simulink model "Monod_Controller"  (R2020b)
settings: Solver=FixedStepAuto  StartTime=0.0  StopTime=constants.tend  FixedStep=constants.dt  RelTol=1e-3
undefined symbols (not defined in the file or in its folder): constants
libraries: pid_lib x2
settings Model: Creator=newpo  LastModifiedBy=newpo
settings DataIOCC: ReturnWorkspaceOutputs=off

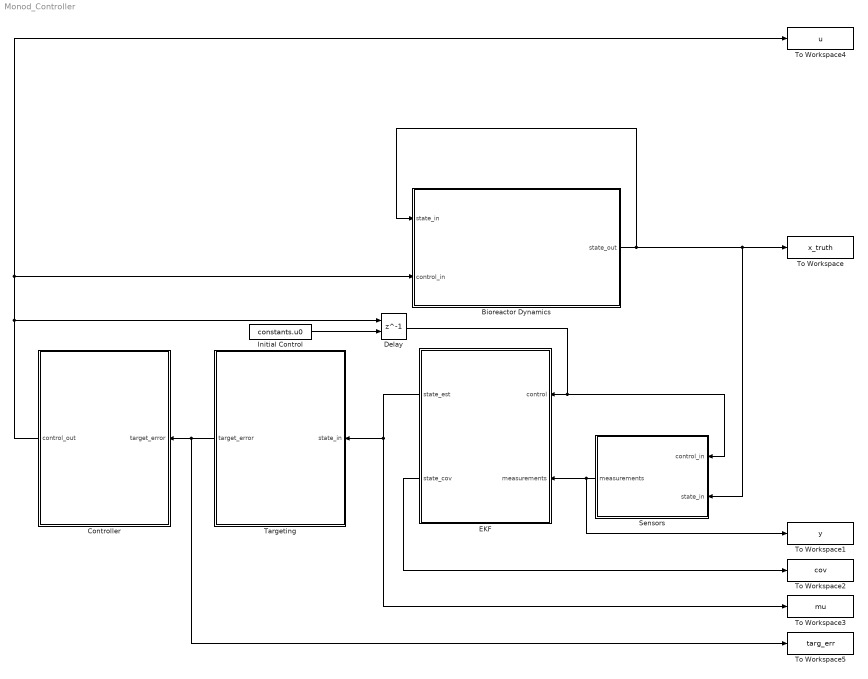
== system Monod_Controller ==
  Bioreactor Dynamics : Subsystem
  Controller : Subsystem
  Delay : Delay  DelayLength=1  InitialConditionSource=Input port  InitialCondition=[constants.w;0;0;constants.Fg]
      settings: InputPortMap=u0,p4
  EKF : Subsystem
  Initial Control : Constant  Value=constants.u0
  Sensors : Subsystem
  Targeting : Subsystem
  To Workspace : ToWorkspace  VariableName=x_truth  SampleTime=-1
  To Workspace1 : ToWorkspace  VariableName=y  SampleTime=-1
  To Workspace2 : ToWorkspace  VariableName=cov  SampleTime=-1
  To Workspace3 : ToWorkspace  VariableName=mu  SampleTime=-1
  To Workspace4 : ToWorkspace  VariableName=u  SampleTime=-1
  To Workspace5 : ToWorkspace  VariableName=targ_err  SampleTime=-1
  wires:
  Bioreactor Dynamics/1(state_out) -> Sensors/2(state_in), To Workspace/1, Bioreactor Dynamics/1(state_in)
  Sensors/1(measurements) -> To Workspace1/1, EKF/2(measurements)
  EKF/1(state_est) -> To Workspace3/1, Targeting/1(state_in)
  Controller/1(control_out) -> To Workspace4/1, Bioreactor Dynamics/2(control_in), Delay/1
  Targeting/1(target_error) -> To Workspace5/1, Controller/1(target_error)
  EKF/2(state_cov) -> To Workspace2/1
  Delay/1 -> Sensors/1(control_in), EKF/1(control)
  Initial Control/1 -> Delay/2

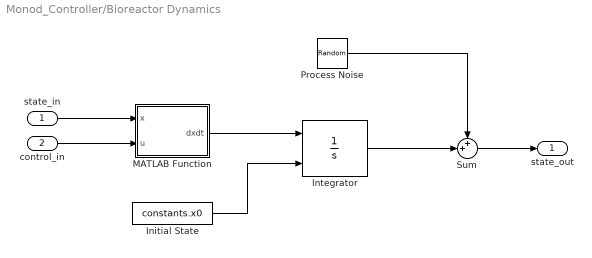
== system Monod_Controller/Bioreactor Dynamics ==
  state_in : Inport
  control_in : Inport  Port=2
  Initial State : Constant  Value=constants.x0
  Integrator : Integrator  InitialConditionSource=external  LimitOutput=on  LowerSaturationLimit=0
  MATLAB Function : MATLAB Function  TreatAsAtomicUnit=on
  Process Noise : RandomNumber  Variance=diag(constants.Q)  SampleTime=constants.dt
  Sum : Sum  Inputs=++|
  state_out : Outport
  wires:
  Initial State/1 -> Integrator/2
  Sum/1 -> state_out/1
  Integrator/1 -> Sum/2
  Process Noise/1 -> Sum/1
  state_in/1 -> MATLAB Function/1(x)
  control_in/1 -> MATLAB Function/2(u)
  MATLAB Function/1(dxdt) -> Integrator/1

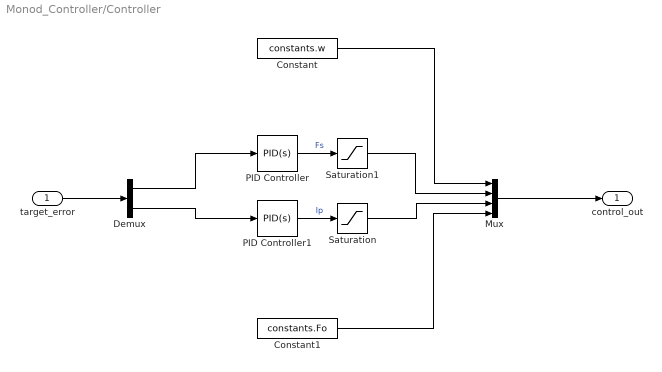
== system Monod_Controller/Controller ==
  target_error : Inport
  Constant : Constant  Value=constants.w
  Constant1 : Constant  Value=constants.Fo
  Demux : Demux  Outputs=2
  Mux : Mux
  PID Controller : pid_lib/PID Controller  Controller=PID  Form=Parallel  TimeDomain=Continuous-time  UseExternalTs=off  SampleTime=-1  IntegratorMethod=Forward Euler  FilterMethod=Forward Euler  ControllerParametersSource=internal  P=1E-3  I=0  D=0  UseFilter=on  N=100  TunerSelectOption=Transfer Function Based (PID Tuner App)  InitialConditionSource=internal  InitialConditionForIntegrator=0  InitialConditionForFilter=0  DifferentiatorICPrevScaledInput=0  ExternalReset=none  TrackingMode=off  Kt=1  LimitOutput=off  SatLimitsSource=internal  UpperSaturationLimit=inf  LowerSaturationLimit=-inf  LinearizeAsGain=on  AntiWindupMode=none  Kb=1  POutMin=[]  POutMax=[]  IOutMin=[]  IOutMax=[]  DOutMin=[]  DOutMax=[]  NOutMin=[]  NOutMax=[]  SumOutMin=[]  SumOutMax=[]  SaturationOutMin=[]  SaturationOutMax=[]  PParamMin=[]  PParamMax=[]  IParamMin=[]  IParamMax=[]  DParamMin=[]  DParamMax=[]  NParamMin=[]  NParamMax=[]  KbParamMin=[]  KbParamMax=[]  KtParamMin=[]  KtParamMax=[]  KbOutMin=[]  KbOutMax=[]  KtOutMin=[]  KtOutMax=[]  IntegratorOutMin=[]  IntegratorOutMax=[]  FilterOutMin=[]  FilterOutMax=[]  SumI1OutMin=[]  SumI1OutMax=[]  SumI2OutMin=[]  SumI2OutMax=[]  SumI3OutMin=[]  SumI3OutMax=[]  SumI4OutMin=[]  SumI4OutMax=[]  SumDOutMin=[]  SumDOutMax=[]  DifferentiatorOutMin=[]  DifferentiatorOutMax=[]  FilterDiffOutCoefMin=[]  FilterDiffOutCoefMax=[]  ReciprocalOutMin=[]  ReciprocalOutMax=[]  SumDenOutMin=[]  SumDenOutMax=[]  SumNumOutMin=[]  SumNumOutMax=[]  DivideOutMin=[]  DivideOutMax=[]  UdiffTsProdOutMin=[]  UdiffTsProdOutMax=[]  NTsProdOutMin=[]  NTsProdOutMax=[]  UintegralTsProdOutMin=[]  UintegralTsProdOutMax=[]  UngainTsProdOutMin=[]  UngainTsProdOutMax=[]  IntegratorContinuousStateAttributes=''  IntegratorStateMustResolveToSignalObject=off  IntegratorRTWStateStorageClass=Auto  FilterContinuousStateAttributes=''  FilterStateMustResolveToSignalObject=off  FilterRTWStateStorageClass=Auto  ParallelPVariant=InternalParameters  IdealPVariant=Disabled  IVariant=InternalParameters  DVariant=InternalParameters  IntegratorVariant=Continuous  SatVariant=Disabled  AWVariant=Passthrough  PCopyVariant=Disabled  TRVariant=Disabled  FdbkBlocksVariant=Forward  IdealPFdbkVariant=Disabled  SatFdbkVariant=Disabled  DerivativeFilterVariant=ContFilter  NVariant=InternalParameters  NCopyVariant=Disabled  FilterICVariant=InternalICsFilter  IntegratorICVariant=InternalICs  ExternalResetVariant=Disabled  TRSumVariant=Passthrough  SumFdbkVariant=Disabled  SumVariant=Sum_PID  TsampFilterVariant=InternalTs  TsampNgainVariant=Passthrough  TsampIntegralVariant=Passthrough  ExternalSaturationOutDataTypeStr=Inherit: Same as second input
  PID Controller1 : pid_lib/PID Controller  Controller=PID  Form=Parallel  TimeDomain=Continuous-time  UseExternalTs=off  SampleTime=-1  IntegratorMethod=Forward Euler  FilterMethod=Forward Euler  ControllerParametersSource=internal  P=8.9545  I=0.12704  D=5.7234  UseFilter=on  N=3  TunerSelectOption=Transfer Function Based (PID Tuner App)  InitialConditionSource=internal  InitialConditionForIntegrator=0  InitialConditionForFilter=0  DifferentiatorICPrevScaledInput=0  ExternalReset=none  TrackingMode=off  Kt=1  LimitOutput=off  SatLimitsSource=internal  UpperSaturationLimit=inf  LowerSaturationLimit=-inf  LinearizeAsGain=on  AntiWindupMode=none  Kb=1  POutMin=[]  POutMax=[]  IOutMin=[]  IOutMax=[]  DOutMin=[]  DOutMax=[]  NOutMin=[]  NOutMax=[]  SumOutMin=[]  SumOutMax=[]  SaturationOutMin=[]  SaturationOutMax=[]  PParamMin=[]  PParamMax=[]  IParamMin=[]  IParamMax=[]  DParamMin=[]  DParamMax=[]  NParamMin=[]  NParamMax=[]  KbParamMin=[]  KbParamMax=[]  KtParamMin=[]  KtParamMax=[]  KbOutMin=[]  KbOutMax=[]  KtOutMin=[]  KtOutMax=[]  IntegratorOutMin=[]  IntegratorOutMax=[]  FilterOutMin=[]  FilterOutMax=[]  SumI1OutMin=[]  SumI1OutMax=[]  SumI2OutMin=[]  SumI2OutMax=[]  SumI3OutMin=[]  SumI3OutMax=[]  SumI4OutMin=[]  SumI4OutMax=[]  SumDOutMin=[]  SumDOutMax=[]  DifferentiatorOutMin=[]  DifferentiatorOutMax=[]  FilterDiffOutCoefMin=[]  FilterDiffOutCoefMax=[]  ReciprocalOutMin=[]  ReciprocalOutMax=[]  SumDenOutMin=[]  SumDenOutMax=[]  SumNumOutMin=[]  SumNumOutMax=[]  DivideOutMin=[]  DivideOutMax=[]  UdiffTsProdOutMin=[]  UdiffTsProdOutMax=[]  NTsProdOutMin=[]  NTsProdOutMax=[]  UintegralTsProdOutMin=[]  UintegralTsProdOutMax=[]  UngainTsProdOutMin=[]  UngainTsProdOutMax=[]  IntegratorContinuousStateAttributes=''  IntegratorStateMustResolveToSignalObject=off  IntegratorRTWStateStorageClass=Auto  FilterContinuousStateAttributes=''  FilterStateMustResolveToSignalObject=off  FilterRTWStateStorageClass=Auto  ParallelPVariant=InternalParameters  IdealPVariant=Disabled  IVariant=InternalParameters  DVariant=InternalParameters  IntegratorVariant=Continuous  SatVariant=Disabled  AWVariant=Passthrough  PCopyVariant=Disabled  TRVariant=Disabled  FdbkBlocksVariant=Forward  IdealPFdbkVariant=Disabled  SatFdbkVariant=Disabled  DerivativeFilterVariant=ContFilter  NVariant=InternalParameters  NCopyVariant=Disabled  FilterICVariant=InternalICsFilter  IntegratorICVariant=InternalICs  ExternalResetVariant=Disabled  TRSumVariant=Passthrough  SumFdbkVariant=Disabled  SumVariant=Sum_PID  TsampFilterVariant=InternalTs  TsampNgainVariant=Passthrough  TsampIntegralVariant=Passthrough  ExternalSaturationOutDataTypeStr=Inherit: Same as second input
  Saturation : Saturate  UpperLimit=constants.Ip_max  LowerLimit=-constants.Ip_max
  Saturation1 : Saturate  UpperLimit=constants.Fs_max  LowerLimit=0
  control_out : Outport
  wires:
  Mux/1 -> control_out/1
  target_error/1 -> Demux/1
  PID Controller/1 -> Saturation1/1  "Fs"
  Demux/1 -> PID Controller/1
  Constant/1 -> Mux/1
  Constant1/1 -> Mux/4
  PID Controller1/1 -> Saturation/1  "Ip"
  Demux/2 -> PID Controller1/1
  Saturation/1 -> Mux/3
  Saturation1/1 -> Mux/2

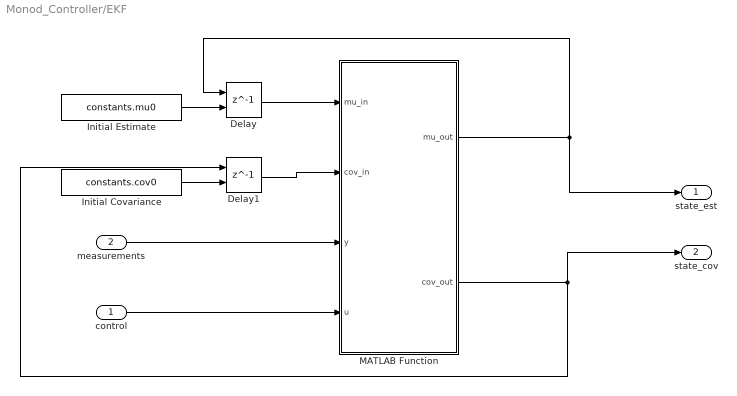
== system Monod_Controller/EKF ==
  control : Inport
  measurements : Inport  Port=2
  Delay : Delay  DelayLength=1  InitialConditionSource=Input port  InitialCondition=0
      settings: InputPortMap=u0,p4
  Delay1 : Delay  DelayLength=1  InitialConditionSource=Input port  InitialCondition=0
      settings: InputPortMap=u0,p4
  Initial Covariance : Constant  Value=constants.cov0
  Initial Estimate : Constant  Value=constants.mu0
  MATLAB Function : MATLAB Function  TreatAsAtomicUnit=on
  state_est : Outport
  state_cov : Outport  Port=2
  wires:
  measurements/1 -> MATLAB Function/3(y)
  Delay/1 -> MATLAB Function/1(mu_in)
  Delay1/1 -> MATLAB Function/2(cov_in)
  Initial Covariance/1 -> Delay1/2
  Initial Estimate/1 -> Delay/2
  MATLAB Function/2(cov_out) -> Delay1/1, state_cov/1
  MATLAB Function/1(mu_out) -> Delay/1, state_est/1
  control/1 -> MATLAB Function/4(u)

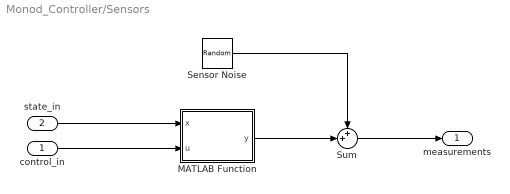
== system Monod_Controller/Sensors ==
  control_in : Inport
  state_in : Inport  Port=2
  MATLAB Function : MATLAB Function  TreatAsAtomicUnit=on
  Sensor Noise : RandomNumber  Variance=diag(constants.R)  SampleTime=constants.dt
  Sum : Sum  Inputs=++|
  measurements : Outport
  wires:
  state_in/1 -> MATLAB Function/1(x)
  control_in/1 -> MATLAB Function/2(u)
  MATLAB Function/1(y) -> Sum/2
  Sum/1 -> measurements/1
  Sensor Noise/1 -> Sum/1

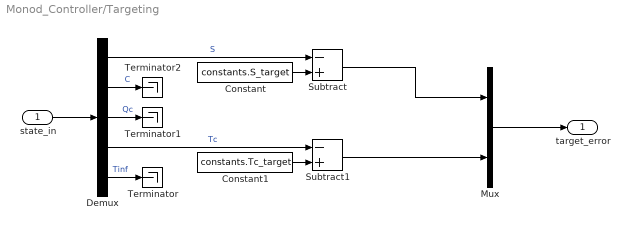
== system Monod_Controller/Targeting ==
  state_in : Inport
  Constant : Constant  Value=constants.S_target
  Constant1 : Constant  Value=constants.Tc_target
  Demux : Demux  Outputs=5
  Mux : Mux  Inputs=2
  Subtract : Sum  Inputs=-+
  Subtract1 : Sum  Inputs=-+
  Terminator : Terminator
  Terminator1 : Terminator
  Terminator2 : Terminator
  target_error : Outport
  wires:
  state_in/1 -> Demux/1
  Demux/5 -> Terminator/1  "Tinf"
  Demux/3 -> Terminator1/1  "Qc"
  Demux/1 -> Subtract/1  "S"
  Demux/4 -> Subtract1/1  "Tc"
  Constant/1 -> Subtract/2
  Constant1/1 -> Subtract1/2
  Subtract/1 -> Mux/1
  Subtract1/1 -> Mux/2
  Mux/1 -> target_error/1
  Demux/2 -> Terminator2/1  "C"

== matlab function Monod_Controller/EKF/MATLAB Function ==
  data: mu_in input; cov_in input; y input; u input; mu_out output; cov_out output; constants parameter
function [mu_out, cov_out] = Monod_EKF(mu_in, cov_in, y, u, constants)
    % Collect inputs
%     S = mu_in(1); % cell concentration, g/l
%     C = mu_in(2); % substrate concentration, g/l
%     QO2 = mu_in(3); % OTR = OUR, moles/sec
%     Tc = mu_in(4); % Temperature of culture
%     Tinf = mu_in(5); % Temperature of environment
    mygrowthrate = mu(mu_in(1),mu_in(2)); 
    
    % Collect controls
    w = u(1); % agitator speed, rpm
    Fs = u(2); % substrate feed rate, L/s
    Ip = u(3); % Peltier current, amps
    Fg = u(4); % air feed rate, SLPS
    kLa = w^(1.7)/(Fg^0.1); % kLa coeff
    
    % Collect measurements
%     mf_out = y(1);
%     DO = y(2);
%     Tc_meas = y(3);
%     Tinf_meas = y(4);
    
    % EKF Update
    mu_p = f(mu_in);
    At = A(mu_in);
    cov_p = At*cov_in*(At.') + constants.Q;
    
    % EKF Prediction
    Ct = C(mu_p);
    ypred = g(mu_p);
    Kt = cov_p*(Ct.')/(Ct*cov_p*(Ct.')+constants.R); % Kalman gain
    mu_out = mu_p + Kt*(y - ypred);
    cov_out = (eye(length(mu_in)) - Kt*Ct)*cov_p;
    
    function xt = f(x)
       xt = zeros(size(x));
       
       xt(1) = x(1) + constants.dt*(constants.S0*Fs/constants.V - Fs/constants.V*x(1) - mygrowthrate/constants.Yxs - constants.m*x(2)); % S = substrate conc
       xt(2) = x(2) + constants.dt*(-Fs/constants.V*x(2) + mygrowthrate); % C = cell conc
       xt(3) = x(3); % QO2 = OUR coefficient
       xt(4) = x(4) + constants.dt/constants.C_heat*(constants.N_power*(w^3)+constants.Kq*x(3)*x(2)+(constants.Pp*Ip+(Ip^2)*constants.Rp)*constants.Np + constants.hA*(x(4)-x(5))); % Tc = culture temp
       xt(5) = x(5); % Tinf = environment temp
    end
    function At = A(x)
        At = zeros(length(x));
        mymu = mu(x(1),x(2));
        dmu = constants.mu_max*x(2)*constants.Ki*(constants.Ki*constants.Ks-(x(1)^2))/((constants.Ki+x(1))^2)/((constants.Ks+x(1))^2);
        At(1,1) = 1 - constants.dt*Fs/constants.V - constants.dt*dmu/constants.Yxs;
        At(1,2) = -constants.dt*mymu - constants.m;
        At(2,1) = constants.dt*dmu;
        At(2,2) = 1 - constants.dt*Fs/constants.V + constants.dt*mymu ;
        At(3,3) = 1;
        At(4,2) = constants.dt/constants.C_heat*constants.Kq*x(3);
        At(4,3) = constants.dt/constants.C_heat*constants.Kq*x(2);
        At(4,4) = 1 + constants.dt/constants.C_heat*constants.hA;
        At(4,5) = -constants.dt/constants.C_heat*constants.hA;
        At(5,5) = 1;
    end
    function ypred = g(x)
        ypred = zeros(4,1);
        ypred(1) = constants.mf_in - x(3)*x(2)/Fg; % Measured mass fraction of O2 leaving system
        ypred(2) = 1 - 1/constants.mf_in*(1/Fg - 1/kLa/constants.pr)*x(3)*x(2); % Measured DO2
        ypred(3) = x(4); % Measured Tc
        ypred(4) = x(5); % measured Tinf
    end
    function Ct = C(x)
       Ct = zeros(4,5);
       Ct(1,2) = -x(3)/Fg;
       Ct(1,3) = -x(2)/Fg;
       Ct(2,2) = -1/constants.mf_in * (1/Fg - 1/constants.pr/kLa)*x(3);
       Ct(2,3) = -1/constants.mf_in * (1/Fg - 1/constants.pr/kLa)*x(2);
       Ct(3,4) = 1;
       Ct(4,5) = 1;
    end
    function mut = mu(S,C)
        mut = constants.mu_max*constants.Ki*S/(constants.Ki+S)/(constants.Ks+S)*C ;
    end
end

== matlab function Monod_Controller/Bioreactor Dynamics/MATLAB Function ==
  data: x input; u input; dxdt output; constants parameter
function dxdt = statedot(x,u,constants)
    dxdt = zeros(size(x));
    w = u(1); % agitator speed
    Fs = u(2); % substrate feed rate
    Ip = u(3); % Peltier currents
    mu = constants.mu_max*x(2)*constants.Ki*x(1)/(constants.Ki+x(1))/(constants.Ks+x(1));
    dxdt(1) = constants.S0*Fs/constants.V - Fs/constants.V*x(1) - mu/constants.Yxs - constants.m*x(2); % S = substrate conc
    dxdt(2) = -Fs/constants.V*x(2) + mu; % C = cell conc
    dxdt(3) = 0; % QO2 = OUR coefficient
    dxdt(4) = 1/constants.C_heat*(constants.N_power*(w^3)+constants.Kq*x(3)*x(2)+(constants.Pp*Ip+(Ip^2)*constants.Rp)*constants.Np + constants.hA*(x(4)-x(5))); % Tc = culture temp
    dxdt(5) = 0; % Tinf = environment temp
end

== matlab function Monod_Controller/Sensors/MATLAB Function ==
  data: x input; u input; y output; constants parameter
function y = g(x,u,constants)
    y = zeros(4,1);
    w = u(1);
    Fg = u(4);
    kLa = (w^1.7)/(Fg^0.1);
    y(1) = constants.mf_in - x(3)*x(2)/Fg; % Measured mass fraction of O2 leaving system
    y(2) = 1 - 1/constants.mf_in*(1/Fg - 1/kLa/constants.pr)*x(3)*x(2); % Measured DO2
    y(3) = x(4); % Measured Tc
    y(4) = x(5); % measured Tinf
end
